simulink subsystem "BMS"  (R2021b)
settings: Solver=VariableStepAuto  StartTime=0.0  StopTime=10.0  RelTol=1e-3
undefined symbols (not defined in the file or in its folder): my_val3, my_val4, my_val5, raptor_xcp_function
libraries: Raptor_lib x4
settings Model: Creator=whamada  LastModifiedBy=whamada

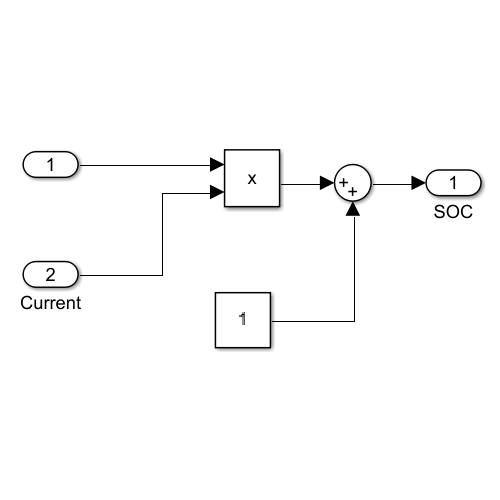
[thumbnail: Simulink's stored preview of the top-level diagram]
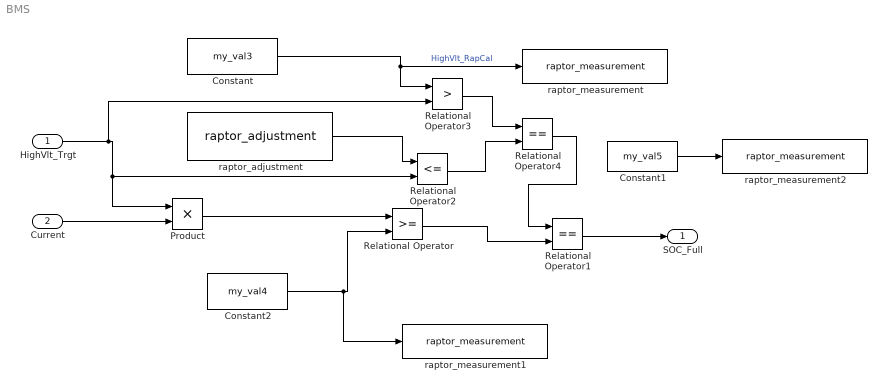
== system BMS ==
  HighVlt_Trgt : Inport  OutDataTypeStr=single  Unit=V  PortDimensions=1
  Current : Inport  Port=2  OutDataTypeStr=single  Unit=ampere  PortDimensions=1
  Constant : Constant  Value=my_val3
  Constant1 : Constant  Value=my_val5
  Constant2 : Constant  Value=my_val4
  Product : Product
  Relational Operator : RelationalOperator  OutDataTypeStr=boolean  RndMeth=Simplest
  Relational Operator1 : RelationalOperator  Operator===  OutDataTypeStr=boolean  RndMeth=Simplest
  Relational Operator2 : RelationalOperator  Operator=<=  OutDataTypeStr=boolean  RndMeth=Simplest
  Relational Operator3 : RelationalOperator  Operator=>  OutDataTypeStr=boolean  RndMeth=Simplest
  Relational Operator4 : RelationalOperator  Operator===  OutDataTypeStr=boolean  RndMeth=Simplest
  raptor_adjustment : Raptor_lib/Data Storage/raptor_adjustment  paramName='CalByRap'  nameSource=Parameter  initValue=33  dataType=double  storage=Calibration  calDispType=Number  calEnum={'False', 'True'}  calGain=1.0  calOffset=0.0  calMax=inf  calMin=-inf  calFormat='-1'  calUnit=''  calHelp=''  calAccess=1  calFunction=raptor_xcp_function(gcb)  calDispHeaders=off  calColHeaders={'Col1' 'Col2' 'Col3'}  calRowHeaders={'Row1' 'Row2' 'Row3'}
      settings: SourceProductName=Raptor
  raptor_measurement : Raptor_lib/Data Storage/raptor_measurement  paramName='my_val3_moni'  nameSource=Parameter  calDispType=Number  calEnum={'False', 'True'}  calGain=1.0  calOffset=0.0  calMax=inf  calMin=-inf  calFormat='-1'  calUnit=''  calHelp=''  calAccess=1  calFunction=raptor_xcp_function(gcb)  calVisible=on
      settings: SourceProductName=Raptor
  raptor_measurement1 : Raptor_lib/Data Storage/raptor_measurement  paramName='my_val4_moni'  nameSource=Parameter  calDispType=Number  calEnum={'False', 'True'}  calGain=1.0  calOffset=0.0  calMax=inf  calMin=-inf  calFormat='-1'  calUnit=''  calHelp=''  calAccess=1  calFunction=raptor_xcp_function(gcb)  calVisible=on
      settings: SourceProductName=Raptor
  raptor_measurement2 : Raptor_lib/Data Storage/raptor_measurement  paramName='my_val5_moni'  nameSource=Parameter  calDispType=Number  calEnum={'False', 'True'}  calGain=1.0  calOffset=0.0  calMax=inf  calMin=-inf  calFormat='-1'  calUnit=''  calHelp=''  calAccess=1  calFunction=raptor_xcp_function(gcb)  calVisible=on
      settings: SourceProductName=Raptor
  SOC_Full : Outport  OutDataTypeStr=boolean  Unit=%  PortDimensions=1
  wires:
  Relational Operator/1 -> Relational Operator1/2
  Constant2/1 -> Relational Operator/2, raptor_measurement1/1
  Current/1 -> Product/2
  Product/1 -> Relational Operator/1
  HighVlt_Trgt/1 -> Product/1, Relational Operator2/2, Relational Operator3/2
  Relational Operator1/1 -> SOC_Full/1
  raptor_adjustment/1 -> Relational Operator2/1
  Constant/1 -> Relational Operator3/1, raptor_measurement/1  "HighVlt_RapCal"
  Relational Operator2/1 -> Relational Operator4/2
  Relational Operator3/1 -> Relational Operator4/1
  Relational Operator4/1 -> Relational Operator1/1
  Constant1/1 -> raptor_measurement2/1
